simulink model "qdrdac"  (R2012b)
(part 2 of 45)

  fftcoefselector/17(timestamp) -> [fftcounter]
  extract_sync_enable_2/4(swts) -> [swtimestamp2bit_1]
  sw_timestamp/1(in_reg) -> [swtimestamp32]
  FIFO64_3/1 -> datamux1/3, [mfifo_q4]
  Counter14/1 -> numdoneevts1/1(out_reg)
  [rst_full_counters] -> Counter14/1
  Counter15/1 -> numdoneevts0/1(out_reg)
  [rst_full_counters] -> Counter15/1
  Counter18/1 -> evtfifordA/1(out_reg)
  [rst_full_counters] -> Counter6/1
  Counter19/1 -> evtfifordB/1(out_reg)
  [rst_full_counters] -> Counter19/1
  Constant3/1 -> sw_timestamp/1(sim_1)
  SigmaDeltaSecOrder/1(DataOut) -> Delay4/1
  Delay4/1 -> sync_out/1
  fifoRdSettingsA/11(Out11) -> [en_ramp_gen]
  [en_ramp_gen] -> Delay4/2
  MCode/6 -> [wr_data_select1]
  MCode2/6 -> [wr_data_sel2]
  MCode2/2 -> [wr_big_fifo2], Counter7/2
  [flushfifo] -> FRD/6(clr_fifos)
  [fsmrst] -> FRD/5(rst)
  [event_length] -> FRD/1(evtlen)
  SinglaEvtFIFO1/2 -> FRD/2(fifo_empty)
  SinglaEvtFIFO1/1 -> FRD/3(data_in)
  [save_event] -> FRD/4(new_evt_rdy)
  FRD/3(out_wr) -> GBEthernet/7(wr1), Counter8/2
  FRD/1(evt_fifo_rd) -> Counter18/2, SinglaEvtFIFO1/3
  fifoRdSettingsA/12(Out12) -> [fluxdemod]
  fifoRdSettingsA/13(Out13) -> [savefluxraw]
  [savefluxraw] -> FRD/8(savefluxraw)
  [fluxdemod] -> FRD/7(isflux_demod)
  [fsmrst] -> FRD1/5(rst)
  [flushfifo] -> FRD1/6(clr_fifos)
  SinglaEvtFIFO2/1 -> FRD1/3(data_in)
  FRD1/1(evt_fifo_rd) -> SinglaEvtFIFO2/3, Counter19/2
  SinglaEvtFIFO2/2 -> FRD1/2(fifo_empty)
  [event_length] -> FRD1/1(evtlen)
  [fluxdemod] -> FRD1/7(isflux_demod)
  [savefluxraw] -> FRD1/8(savefluxraw)
  FRD1/3(out_wr) -> GBEthernet/10(wr2), Counter9/2
  Counter20/1 -> chanFifoFull2/1(out_reg)
  FIFO64_1/6 -> Counter20/2
  [rst_full_counters] -> Counter20/1
  Counter21/1 -> chanFifoFull3/1(out_reg)
  FIFO64_3/6 -> Counter21/2
  [savetranslated] -> FRD/9(circletrans)
  [savetranslated] -> FRD1/9(circletrans)
  RampTiming/1(synctofft) -> [syncsave]
  [rst_full_counters] -> RampTiming/1(rstcnt)
  sw_timestamp2/1(in_reg) -> RampTiming/2(swts2)
  [fft_coef_sync] -> RampTiming/3(fftcoefsync)
  syncDelay/1(in_reg) -> RampTiming/4(syncdelay)
  Mux/1 -> RampTiming/5(sync)
  RampTiming/2(numsync1) -> numSyncPulses1/1(out_reg)
  RampTiming/3(numsync) -> numSyncPulses/1(out_reg)
  fftcoefselector/12(fftshiftx) -> WindowAndFFT/1(In1)
  fftcoefselector/15(stopfft) -> WindowAndFFT/3(In3)
  WindowAndFFT/2(Out6) -> FineMix/9(In9), Delay31/1
  WindowAndFFT/4(Out8) -> FineMix/11(In12), Delay33/1
  WindowAndFFT/5(Out9) -> FineMix/12(In13), Delay34/1
  WindowAndFFT/1(Out5) -> fftcoefselector/1(fftsyncout)
  WindowAndFFT/3(Out7) -> FineMix/10(In11), Delay32/1
  FineMix/9(dvldout4) -> FIFO64_3/2, Counter5/2
  FineMix/7(dvldout3) -> FIFO64_1/2, Counter4/2
  FineMix/5(dvalout2) -> FIFO64_2/2, Counter3/2
  FineMix/12(dout4) -> Concat/2
  FineMix/10(dout3) -> Concat4/2
  FineMix/6(dout2) -> Concat2/2
  FineMix/3(dout1) -> Concat3/2
  fftcoefselector/2(we0) -> FineMix/1(In1)
  fftcoefselector/3(we1) -> FineMix/2(In2)
  fftcoefselector/4(we2) -> FineMix/3(In3)
  fftcoefselector/5(we3) -> FineMix/4(In4)
  fftcoefselector/6(chan0) -> FineMix/5(In5)
  fftcoefselector/7(chan1) -> FineMix/6(In6)
  fftcoefselector/8(chan2) -> FineMix/7(In7)
  fftcoefselector/9(chan3) -> FineMix/8(In8)
  [start_fft_sync] -> FineMix/13(In16)
  FineMix/1(chanout1) -> FIFO64_4/1
  FineMix/4(chanout2) -> FIFO64_2/1
  FineMix/8(chanout3) -> FIFO64_1/1
  FineMix/11(chanout4) -> FIFO64_3/1
  FIFO64_2/4 -> Terminator5/1
  FIFO64_2/5 -> Terminator6/1
  FIFO64_2/6 -> Terminator7/1
  FIFO64_2/7 -> Terminator8/1
  FIFO64_2/9 -> Terminator9/1
  FIFO64_4/4 -> Terminator/1
  FIFO64_4/5 -> Terminator1/1
  FIFO64_4/6 -> Terminator2/1
  FIFO64_4/7 -> Terminator3/1
  FIFO64_4/9 -> Terminator4/1
  zero_bool_1/1 -> FIFO64_2/8, FIFO64_2/7
  zero_bool_2/1 -> FIFO64_1/8, FIFO64_1/7
  zero_bool_4/1 -> FIFO64_3/7, FIFO64_3/8
  Counter2/1 -> fifowrA/1(out_reg)
  FineMix/2(dvalout1) -> Counter2/2, FIFO64_4/2
  sync_bit2/1 -> roachscope/4(In4)
  sync_bit3/1 -> roachscope/5(In5)
  sync_bit4/1 -> roachscope/6(In6)
  sync_bit5/1 -> roachscope/7(In7)
  sync_bit6/1 -> roachscope/8(In8)
  fifoRdSettingsA/14(Out14) -> [savetranslated]
  [dumpfifo] -> MCode/1
  [fsmrst] -> MCode/4
  [is_look_sync] -> MCode/11
  [flushfifo] -> MCode/8
  [rst_full_counters] -> Counter2/1
  [syncsave] -> Concat/1
  [syncsave] -> Concat4/1
  [syncsave] -> Concat2/1
  [syncsave] -> Concat3/1
  [syncsave] -> roachscope/3(In3)
  [rst_full_counters] -> Counter5/1
  [muxsel_a] -> vldmux/1
  [muxsel_a] -> quartfull/1
  [muxsel_a] -> emptymux/1
  [muxsel_a] -> datamux/1
  [event_length] -> MCode/9
  [event_length] -> MCode2/9
  readFifoSize/1(in_reg) -> [event_length]
  [last_channel] -> MCode/6
  [last_channel] -> MCode2/6
  [current_chan1] -> extract_sync_enable_2/3(chan)
  [current_chan1] -> dataformatter2/2(channel_)
  [current_chan1] -> roachscope/2(In2)
  [wr_big_fifo1] -> SinglaEvtFIFO1/2
  MCode/2 -> Counter6/2, [wr_big_fifo1]
  [swtimestamp2bit_1] -> roachscope/1(In1)
  [wr_data_select1] -> dataformatter2/5(wr_data_sel)
  [mfifo_q1] -> sync_bit3/1
  [mfifo_q2] -> sync_bit4/1
  [mfifo_q3] -> sync_bit5/1
  [mfifo_q4] -> sync_bit6/1
  sync_bit/1 -> Delay42/1
  [swtimestamp32] -> dataformatter2/1(timestamp32_)
  [swtimestamp32] -> dataformatter1/1(timestamp32_)
  MCode/1 -> fifoCtrlLogic1/1(In1)
  fifoCtrlLogic1/1(Out1) -> [fiford0]
  fifoCtrlLogic1/2(Out2) -> [fiford1]
  fifoCtrlLogic1/3(Out3) -> [muxsel_a]
  fifoCtrlLogic1/4(Out4) -> [rdchan_a]
  [rst_full_counters] -> Counter18/1
  [current_chan2] -> extract_sync_enable_1/3(chan)
  [current_chan2] -> dataformatter1/2(channel_)
  MCode2/1 -> fifoCtrl2/1(In1)
  fifoCtrl2/1(Out1) -> [fiford2]
  fifoCtrl2/2(Out2) -> [fiford3]
  fifoCtrl2/3(Out3) -> [muxsel_b]
  fifoCtrl2/4(Out4) -> [rdchan_b]
  MCode2/7 -> [save_event2], Counter14/2
  [save_event2] -> FRD1/4(new_evt_rdy)
  [wr_data_sel2] -> dataformatter1/5(wr_data_sel)
  [wr_big_fifo2] -> SinglaEvtFIFO2/2
  [ethernet_rst] -> GBEthernet/1(rstgbe)
  [fsmrst] -> GBEthernet/2(rstfsm)
  [flushfifo] -> GBEthernet/3(clrfifo)
  txdestip/1(in_reg) -> GBEthernet/4(destip)
  txdestport/1(in_reg) -> GBEthernet/5(destport)
  FRD/2(dataout) -> GBEthernet/6(din1)
  [rst_full_counters] -> GBEthernet/8(rst)
  FRD1/2(dataout) -> GBEthernet/9(din2)
  GBEthernet/1(numtxeof) -> gbeofcount/1(out_reg)
  GBEthernet/3(numtxovf) -> gbtxovfcnt/1(out_reg)
  GBEthernet/6(numtxvld) -> gbdatalen/1(out_reg)
  GBEthernet/7(numfiford) -> outfifordA/1(out_reg)
  GBEthernet/10(numrd2) -> outfifordB/1(out_reg)
  Constant1/1 -> txdestport/1(sim_1), txdestip/1(sim_1)
